simulink model "question5sigma"  (R2022b)
settings: Solver=ode4  StartTime=0.0  StopTime=10  FixedStep=0.0001  MaxStep=0.0001  RelTol=1e-3
values from neighbouring files (symbols this model uses):
  A = [a-b, 0.5-c; 0, 1]    [A2_1_2_graph.m]    (also in A2_1_2_val.m; A2_4_1.m = [a-bl, 0.5-c; 0, 1]; A2_4_3.m = [a-bl, 0.5-c; 0, 1]; A2_4_31.m = [a-bl, 0.5-c; 0, 1])
  B = [0; 1]    [A2_1_2_graph.m]    (also in A2_1_2_val.m; A2_4_1.m; A2_4_3.m; A2_4_31.m)
  C = eye(2)    [A2_5_1.m]
  D = zeros(2,1)    [A2_5_1.m]
settings Model: Creator=long  LastModifiedBy=munjunhwi
settings SolverCC: AlgebraicLoopSolver=TrustRegion
settings DebuggingCC: UnconnectedInputMsg=warning  UnconnectedOutputMsg=warning  UnconnectedLineMsg=warning  SFMachineParentedDataDiag=warning
settings ModelReferenceCC: EnableRefExpFcnMdlSchedulingChecks=on
settings RTWCC: DLArmComputeVersion=19.05

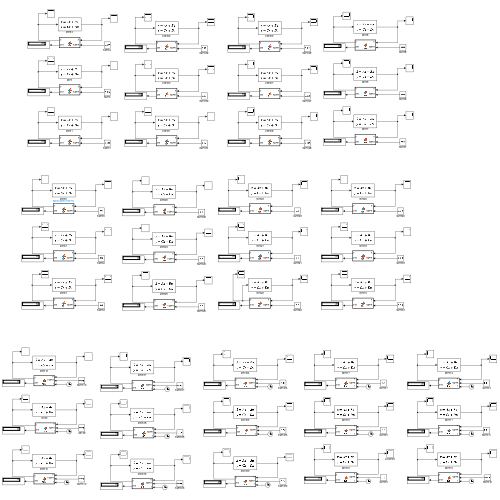
[thumbnail: Simulink's stored preview of the top-level diagram]
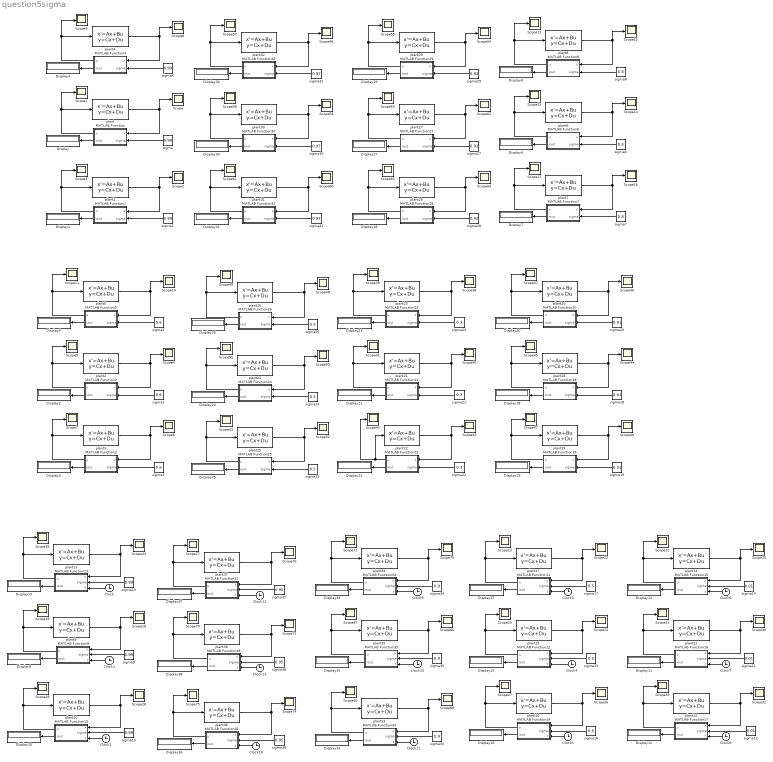
== system question5sigma ==
  Clock{,1..14} (15 alike) : Clock
  Display{,1..38} (39 alike) : Display
  MATLAB Function : MATLAB Function  TreatAsAtomicUnit=on
  MATLAB Function1 : MATLAB Function  TreatAsAtomicUnit=on
  MATLAB Function10 : MATLAB Function  TreatAsAtomicUnit=on
  MATLAB Function11 : MATLAB Function  TreatAsAtomicUnit=on
  MATLAB Function12 : MATLAB Function  TreatAsAtomicUnit=on
  MATLAB Function13 : MATLAB Function  TreatAsAtomicUnit=on
  MATLAB Function14 : MATLAB Function  TreatAsAtomicUnit=on
  MATLAB Function15 : MATLAB Function  TreatAsAtomicUnit=on
  MATLAB Function16 : MATLAB Function  TreatAsAtomicUnit=on
  MATLAB Function17 : MATLAB Function  TreatAsAtomicUnit=on
  MATLAB Function18 : MATLAB Function  TreatAsAtomicUnit=on
  MATLAB Function19 : MATLAB Function  TreatAsAtomicUnit=on
  MATLAB Function2 : MATLAB Function  TreatAsAtomicUnit=on
  MATLAB Function20 : MATLAB Function  TreatAsAtomicUnit=on
  MATLAB Function21 : MATLAB Function  TreatAsAtomicUnit=on
  MATLAB Function22 : MATLAB Function  TreatAsAtomicUnit=on
  MATLAB Function23 : MATLAB Function  TreatAsAtomicUnit=on
  MATLAB Function24 : MATLAB Function  TreatAsAtomicUnit=on
  MATLAB Function25 : MATLAB Function  TreatAsAtomicUnit=on
  MATLAB Function26 : MATLAB Function  TreatAsAtomicUnit=on
  MATLAB Function27 : MATLAB Function  TreatAsAtomicUnit=on
  MATLAB Function28 : MATLAB Function  TreatAsAtomicUnit=on
  MATLAB Function29 : MATLAB Function  TreatAsAtomicUnit=on
  MATLAB Function3 : MATLAB Function  TreatAsAtomicUnit=on
  MATLAB Function30 : MATLAB Function  TreatAsAtomicUnit=on
  MATLAB Function31 : MATLAB Function  TreatAsAtomicUnit=on
  MATLAB Function32 : MATLAB Function  TreatAsAtomicUnit=on
  MATLAB Function33 : MATLAB Function  TreatAsAtomicUnit=on
  MATLAB Function34 : MATLAB Function  TreatAsAtomicUnit=on
  MATLAB Function35 : MATLAB Function  TreatAsAtomicUnit=on
  MATLAB Function36 : MATLAB Function  TreatAsAtomicUnit=on
  MATLAB Function37 : MATLAB Function  TreatAsAtomicUnit=on
  MATLAB Function38 : MATLAB Function  TreatAsAtomicUnit=on
  MATLAB Function4 : MATLAB Function  TreatAsAtomicUnit=on
  MATLAB Function5 : MATLAB Function  TreatAsAtomicUnit=on
  MATLAB Function6 : MATLAB Function  TreatAsAtomicUnit=on
  MATLAB Function7 : MATLAB Function  TreatAsAtomicUnit=on
  MATLAB Function8 : MATLAB Function  TreatAsAtomicUnit=on
  MATLAB Function9 : MATLAB Function  TreatAsAtomicUnit=on
  Scope{,1..77} (78 alike) : Scope
  plant{,2,6,9,11,15,18,21,24,27,30,35,38} (13 alike) : StateSpace  A=A  B=B  C=C  D=D  InitialCondition=[10;10]
  plant{1,3,7,10,12,16,19,22,25,28,31,33,36} (13 alike) : StateSpace  A=A  B=B  C=C  D=D  InitialCondition=[1;0]
  plant{4..5,8,13..14,17,20,23,26,29,32,34,37} (13 alike) : StateSpace  A=A  B=B  C=C  D=D  InitialCondition=[100;150]
  sigma{,1,4,9..10,13} (6 alike) : Constant  Value=0.99
  sigma{11..12,14,18..20} (6 alike) : Constant  Value=0.01
  sigma{15..17,24..26} (6 alike) : Constant  Value=0.5
  sigma2 : Constant  Value=0.6
  sigma21 : Constant  Value=0.3
  sigma22 : Constant  Value=0.3
  sigma23 : Constant  Value=0.3
  sigma27 : Constant  Value=0.92
  sigma28 : Constant  Value=0.92
  sigma29 : Constant  Value=0.92
  sigma3 : Constant  Value=0.6
  sigma30 : Constant  Value=0.97
  sigma31 : Constant  Value=0.97
  sigma32 : Constant  Value=0.97
  sigma33 : Constant  Value=0.9
  sigma34 : Constant  Value=0.9
  sigma35 : Constant  Value=0.9
  sigma36 : Constant  Value=0.95
  sigma37 : Constant  Value=0.95
  sigma38 : Constant  Value=0.95
  sigma5 : Constant  Value=0.6
  sigma6 : Constant  Value=0.8
  sigma7 : Constant  Value=0.8
  sigma8 : Constant  Value=0.8
  wires:
  sigma/1 -> MATLAB Function/2(sigma)
  plant/1 -> MATLAB Function/1(x), Scope/1
  MATLAB Function/1(u) -> Scope1/1, plant/1
  MATLAB Function/2(iout) -> Display/1
  MATLAB Function1/2(iout) -> Display1/1
  MATLAB Function1/1(u) -> Scope3/1, plant1/1
  sigma1/1 -> MATLAB Function1/2(sigma)
  plant1/1 -> MATLAB Function1/1(x), Scope2/1
  MATLAB Function2/2(iout) -> Display2/1
  MATLAB Function2/1(u) -> Scope5/1, plant2/1
  sigma2/1 -> MATLAB Function2/2(sigma)
  plant2/1 -> MATLAB Function2/1(x), Scope4/1
  MATLAB Function3/2(iout) -> Display3/1
  MATLAB Function3/1(u) -> Scope7/1, plant3/1
  sigma3/1 -> MATLAB Function3/2(sigma)
  plant3/1 -> MATLAB Function3/1(x), Scope6/1
  sigma5/1 -> MATLAB Function5/2(sigma)
  MATLAB Function5/1(u) -> Scope11/1, plant5/1
  MATLAB Function4/2(iout) -> Display4/1
  MATLAB Function4/1(u) -> Scope9/1, plant4/1
  sigma4/1 -> MATLAB Function4/2(sigma)
  plant5/1 -> MATLAB Function5/1(x), Scope10/1
  MATLAB Function5/2(iout) -> Display5/1
  plant4/1 -> MATLAB Function4/1(x), Scope8/1
  sigma6/1 -> MATLAB Function6/2(sigma)
  MATLAB Function6/1(u) -> Scope15/1, plant6/1
  plant6/1 -> MATLAB Function6/1(x), Scope14/1
  MATLAB Function8/1(u) -> Scope13/1, plant8/1
  MATLAB Function8/2(iout) -> Display8/1
  plant8/1 -> MATLAB Function8/1(x), Scope12/1
  MATLAB Function6/2(iout) -> Display6/1
  sigma8/1 -> MATLAB Function8/2(sigma)
  sigma7/1 -> MATLAB Function7/2(sigma)
  MATLAB Function7/1(u) -> Scope17/1, plant7/1
  plant7/1 -> MATLAB Function7/1(x), Scope16/1
  MATLAB Function7/2(iout) -> Display7/1
  sigma11/1 -> MATLAB Function16/2(sigma)
  MATLAB Function16/1(u) -> Scope31/1, plant11/1
  plant11/1 -> MATLAB Function16/1(x), Scope30/1
  MATLAB Function10/2(iout) -> Display10/1
  sigma10/1 -> MATLAB Function10/2(sigma)
  plant10/1 -> MATLAB Function10/1(x), Scope28/1
  MATLAB Function15/1(u) -> Scope21/1, plant14/1
  MATLAB Function13/2(iout) -> Display13/1
  MATLAB Function13/1(u) -> Scope35/1, plant13/1
  plant14/1 -> MATLAB Function15/1(x), Scope20/1
  MATLAB Function16/2(iout) -> Display11/1
  MATLAB Function17/1(u) -> Scope33/1, plant12/1
  sigma12/1 -> MATLAB Function17/2(sigma)
  MATLAB Function17/2(iout) -> Display12/1
  plant12/1 -> MATLAB Function17/1(x), Scope32/1
  MATLAB Function14/2(iout) -> Display16/1
  plant16/1 -> MATLAB Function14/1(x), Scope26/1
  MATLAB Function12/2(iout) -> Display15/1
  sigma16/1 -> MATLAB Function14/2(sigma)
  plant17/1 -> MATLAB Function11/1(x), Scope22/1
  sigma14/1 -> MATLAB Function15/2(sigma)
  MATLAB Function14/1(u) -> Scope27/1, plant16/1
  MATLAB Function10/1(u) -> Scope29/1, plant10/1
  plant15/1 -> MATLAB Function12/1(x), Scope24/1
  MATLAB Function12/1(u) -> Scope25/1, plant15/1
  sigma13/1 -> MATLAB Function13/2(sigma)
  MATLAB Function11/2(iout) -> Display17/1
  MATLAB Function11/1(u) -> Scope23/1, plant17/1
  sigma17/1 -> MATLAB Function11/2(sigma)
  MATLAB Function9/1(u) -> Scope19/1, plant9/1
  MATLAB Function9/2(iout) -> Display9/1
  MATLAB Function15/2(iout) -> Display14/1
  sigma9/1 -> MATLAB Function9/2(sigma)
  plant9/1 -> MATLAB Function9/1(x), Scope18/1
  sigma15/1 -> MATLAB Function12/2(sigma)
  plant13/1 -> MATLAB Function13/1(x), Scope34/1
  Clock/1 -> MATLAB Function13/3(t)
  Clock1/1 -> MATLAB Function9/3(t)
  Clock2/1 -> MATLAB Function10/3(t)
  Clock3/1 -> MATLAB Function11/3(t)
  Clock4/1 -> MATLAB Function12/3(t)
  Clock5/1 -> MATLAB Function14/3(t)
  Clock6/1 -> MATLAB Function15/3(t)
  Clock7/1 -> MATLAB Function16/3(t)
  Clock8/1 -> MATLAB Function17/3(t)
  MATLAB Function18/2(iout) -> Display18/1
  MATLAB Function23/1(u) -> Scope39/1, plant23/1
  MATLAB Function22/2(iout) -> Display22/1
  MATLAB Function22/1(u) -> Scope43/1, plant22/1
  sigma22/1 -> MATLAB Function22/2(sigma)
  MATLAB Function23/2(iout) -> Display23/1
  sigma20/1 -> MATLAB Function20/2(sigma)
  plant23/1 -> MATLAB Function23/1(x), Scope38/1
  sigma23/1 -> MATLAB Function23/2(sigma)
  MATLAB Function19/2(iout) -> Display19/1
  MATLAB Function18/1(u) -> Scope45/1, plant18/1
  sigma18/1 -> MATLAB Function18/2(sigma)
  MATLAB Function20/1(u) -> Scope37/1, plant20/1
  plant18/1 -> MATLAB Function18/1(x), Scope44/1
  MATLAB Function20/2(iout) -> Display20/1
  plant20/1 -> MATLAB Function20/1(x), Scope36/1
  plant21/1 -> MATLAB Function21/1(x), Scope40/1
  MATLAB Function21/2(iout) -> Display21/1
  MATLAB Function21/1(u) -> Scope41/1, plant21/1
  plant19/1 -> MATLAB Function19/1(x), Scope46/1
  MATLAB Function19/1(u) -> Scope47/1, plant19/1
  plant22/1 -> MATLAB Function22/1(x), Scope42/1
  sigma19/1 -> MATLAB Function19/2(sigma)
  sigma21/1 -> MATLAB Function21/2(sigma)
  MATLAB Function26/1(u) -> Scope49/1, plant26/1
  MATLAB Function25/1(u) -> Scope53/1, plant25/1
  MATLAB Function24/2(iout) -> Display24/1
  sigma26/1 -> MATLAB Function26/2(sigma)
  sigma25/1 -> MATLAB Function25/2(sigma)
  plant26/1 -> MATLAB Function26/1(x), Scope48/1
  MATLAB Function26/2(iout) -> Display26/1
  MATLAB Function24/1(u) -> Scope51/1, plant24/1
  plant24/1 -> MATLAB Function24/1(x), Scope50/1
  MATLAB Function25/2(iout) -> Display25/1
  plant25/1 -> MATLAB Function25/1(x), Scope52/1
  sigma24/1 -> MATLAB Function24/2(sigma)
  MATLAB Function27/2(iout) -> Display27/1
  MATLAB Function32/1(u) -> Scope57/1, plant32/1
  MATLAB Function31/2(iout) -> Display31/1
  MATLAB Function31/1(u) -> Scope61/1, plant31/1
  sigma31/1 -> MATLAB Function31/2(sigma)
  MATLAB Function32/2(iout) -> Display32/1
  sigma29/1 -> MATLAB Function29/2(sigma)
  plant32/1 -> MATLAB Function32/1(x), Scope56/1
  sigma32/1 -> MATLAB Function32/2(sigma)
  MATLAB Function28/2(iout) -> Display28/1
  MATLAB Function27/1(u) -> Scope63/1, plant27/1
  sigma27/1 -> MATLAB Function27/2(sigma)
  MATLAB Function29/1(u) -> Scope55/1, plant29/1
  plant27/1 -> MATLAB Function27/1(x), Scope62/1
  MATLAB Function29/2(iout) -> Display29/1
  plant29/1 -> MATLAB Function29/1(x), Scope54/1
  plant30/1 -> MATLAB Function30/1(x), Scope58/1
  MATLAB Function30/2(iout) -> Display30/1
  MATLAB Function30/1(u) -> Scope59/1, plant30/1
  plant28/1 -> MATLAB Function28/1(x), Scope64/1
  MATLAB Function28/1(u) -> Scope65/1, plant28/1
  plant31/1 -> MATLAB Function31/1(x), Scope60/1
  sigma28/1 -> MATLAB Function28/2(sigma)
  sigma30/1 -> MATLAB Function30/2(sigma)
  MATLAB Function33/2(iout) -> Display33/1
  sigma33/1 -> MATLAB Function33/2(sigma)
  MATLAB Function35/2(iout) -> Display35/1
  MATLAB Function33/1(u) -> Scope69/1, plant33/1
  plant35/1 -> MATLAB Function35/1(x), Scope66/1
  MATLAB Function35/1(u) -> Scope67/1, plant35/1
  sigma34/1 -> MATLAB Function34/2(sigma)
  MATLAB Function34/2(iout) -> Display34/1
  sigma35/1 -> MATLAB Function35/2(sigma)
  MATLAB Function34/1(u) -> Scope71/1, plant34/1
  plant33/1 -> MATLAB Function33/1(x), Scope68/1
  plant34/1 -> MATLAB Function34/1(x), Scope70/1
  Clock9/1 -> MATLAB Function34/3(t)
  Clock10/1 -> MATLAB Function35/3(t)
  Clock11/1 -> MATLAB Function33/3(t)
  MATLAB Function36/2(iout) -> Display36/1
  sigma36/1 -> MATLAB Function36/2(sigma)
  MATLAB Function38/2(iout) -> Display38/1
  MATLAB Function36/1(u) -> Scope75/1, plant36/1
  plant38/1 -> MATLAB Function38/1(x), Scope72/1
  MATLAB Function38/1(u) -> Scope73/1, plant38/1
  sigma37/1 -> MATLAB Function37/2(sigma)
  MATLAB Function37/2(iout) -> Display37/1
  sigma38/1 -> MATLAB Function38/2(sigma)
  MATLAB Function37/1(u) -> Scope77/1, plant37/1
  plant36/1 -> MATLAB Function36/1(x), Scope74/1
  plant37/1 -> MATLAB Function37/1(x), Scope76/1
  Clock12/1 -> MATLAB Function37/3(t)
  Clock13/1 -> MATLAB Function38/3(t)
  Clock14/1 -> MATLAB Function36/3(t)

== matlab function question5sigma/MATLAB Function10 ==
  settings: updateMethod=DISCRETE
  data: x input; u output; sigma input; iout output; t input
function [u,iout]= fcn(x,sigma,t)
    persistent uk xk i;
    k1=zeros(1,2);
    A=zeros(2);
    B=zeros(2,1);
    P=zeros(2);
    Q=zeros(2);
    coder.extrinsic('evalin');
    A = evalin('base', 'A'); 
    B = evalin('base', 'B'); 
    P = evalin('base', 'P'); 
    Q = evalin('base', 'Q'); 
    k1 = evalin('base', 'k1'); 
    
    
    if isempty(uk)||isempty(xk)
        i=0;
        xk = x;
        uk=-k1*x;
    end

    
    if rem(t,0.2174)==0
        if [x' xk']*[A'*P+P*A+sigma*Q -P*B*k1;-(B*k1)'*P zeros(2)]*[x;xk]>=0
            i = i+1;
            uk = -k1*x;
            xk = x;
        end
    end

    u=uk;
    iout=i;
end

== matlab function question5sigma/MATLAB Function11 ==
  settings: updateMethod=DISCRETE
  data: x input; u output; sigma input; iout output; t input
function [u,iout]= fcn(x,sigma,t)
    persistent uk xk i;
    k1=zeros(1,2);
    A=zeros(2);
    B=zeros(2,1);
    P=zeros(2);
    Q=zeros(2);
    coder.extrinsic('evalin');
    A = evalin('base', 'A'); 
    B = evalin('base', 'B'); 
    P = evalin('base', 'P'); 
    Q = evalin('base', 'Q'); 
    k1 = evalin('base', 'k1'); 
    
    
    if isempty(uk)||isempty(xk)
        i=0;
        xk = x;
        uk=-k1*x;
    end

    
    if rem(t,0.2174)==0
        if [x' xk']*[A'*P+P*A+sigma*Q -P*B*k1;-(B*k1)'*P zeros(2)]*[x;xk]>=0
            i = i+1;
            uk = -k1*x;
            xk = x;
        end
    end

    u=uk;
    iout=i;
end

== matlab function question5sigma/MATLAB Function13 ==
  settings: updateMethod=DISCRETE
  data: x input; u output; sigma input; iout output; t input
function [u,iout]= fcn(x,sigma,t)
    persistent uk xk i;
    k1=zeros(1,2);
    A=zeros(2);
    B=zeros(2,1);
    P=zeros(2);
    Q=zeros(2);
    coder.extrinsic('evalin');
    A = evalin('base', 'A'); 
    B = evalin('base', 'B'); 
    P = evalin('base', 'P'); 
    Q = evalin('base', 'Q'); 
    k1 = evalin('base', 'k1'); 
    
    
    if isempty(uk)||isempty(xk)
        i=0;
        xk = x;
        uk=-k1*x;
    end

    
    if rem(t,0.2174)==0 %sampling time 0.0035
        if [x' xk']*[A'*P+P*A+sigma*Q -P*B*k1;-(B*k1)'*P zeros(2)]*[x;xk]>=0
            i = i+1;
            uk = -k1*x;
            xk = x;
        end
    end

    u=uk;
    iout=i;
end

== matlab function question5sigma/MATLAB Function12 ==
  settings: updateMethod=DISCRETE
  data: x input; u output; sigma input; iout output; t input
function [u,iout]= fcn(x,sigma,t)
    persistent uk xk i;
    k1=zeros(1,2);
    A=zeros(2);
    B=zeros(2,1);
    P=zeros(2);
    Q=zeros(2);
    coder.extrinsic('evalin');
    A = evalin('base', 'A'); 
    B = evalin('base', 'B'); 
    P = evalin('base', 'P'); 
    Q = evalin('base', 'Q'); 
    k1 = evalin('base', 'k1'); 
    
    
    if isempty(uk)||isempty(xk)
        i=0;
        xk = x;
        uk=-k1*x;
    end

    
    if rem(t,0.2174)==0
        if [x' xk']*[A'*P+P*A+sigma*Q -P*B*k1;-(B*k1)'*P zeros(2)]*[x;xk]>=0
            i = i+1;
            uk = -k1*x;
            xk = x;
        end
    end

    u=uk;
    iout=i;
end

== matlab function question5sigma/MATLAB Function14 ==
  settings: updateMethod=DISCRETE
  data: x input; u output; sigma input; iout output; t input
function [u,iout]= fcn(x,sigma,t)
    persistent uk xk i;
    k1=zeros(1,2);
    A=zeros(2);
    B=zeros(2,1);
    P=zeros(2);
    Q=zeros(2);
    coder.extrinsic('evalin');
    A = evalin('base', 'A'); 
    B = evalin('base', 'B'); 
    P = evalin('base', 'P'); 
    Q = evalin('base', 'Q'); 
    k1 = evalin('base', 'k1'); 
    
    
    if isempty(uk)||isempty(xk)
        i=0;
        xk = x;
        uk=-k1*x;
    end

    
    if rem(t,0.2174)==0
        if [x' xk']*[A'*P+P*A+sigma*Q -P*B*k1;-(B*k1)'*P zeros(2)]*[x;xk]>=0
            i = i+1;
            uk = -k1*x;
            xk = x;
        end
    end

    u=uk;
    iout=i;
end

== matlab function question5sigma/MATLAB Function15 ==
  settings: updateMethod=DISCRETE
  data: x input; u output; sigma input; iout output; t input
function [u,iout]= fcn(x,sigma,t)
    persistent uk xk i;
    k1=zeros(1,2);
    A=zeros(2);
    B=zeros(2,1);
    P=zeros(2);
    Q=zeros(2);
    coder.extrinsic('evalin');
    A = evalin('base', 'A'); 
    B = evalin('base', 'B'); 
    P = evalin('base', 'P'); 
    Q = evalin('base', 'Q'); 
    k1 = evalin('base', 'k1'); 
    
    
    if isempty(uk)||isempty(xk)
        i=0;
        xk = x;
        uk=-k1*x;
    end

    
    if rem(t,0.2174)==0
        if [x' xk']*[A'*P+P*A+sigma*Q -P*B*k1;-(B*k1)'*P zeros(2)]*[x;xk]>=0
            i = i+1;
            uk = -k1*x;
            xk = x;
        end
    end

    u=uk;
    iout=i;
end

== matlab function question5sigma/MATLAB Function1 ==
  settings: updateMethod=DISCRETE
  data: x input; u output; sigma input; iout output
function [u,iout]= fcn(x,sigma)
    persistent uk xk i;
    k1=zeros(1,2);
    A=zeros(2);
    B=zeros(2,1);
    P=zeros(2);
    Q=zeros(2);
    coder.extrinsic('evalin');
    A = evalin('base', 'A'); 
    B = evalin('base', 'B'); 
    P = evalin('base', 'P'); 
    Q = evalin('base', 'Q'); 
    k1 = evalin('base', 'k1'); 
    
    
    if isempty(uk)||isempty(xk)
        i=0;
        xk = x;
        uk=-k1*x;
    end

    if [x' xk']*[A'*P+P*A+sigma*Q -P*B*k1;-(B*k1)'*P zeros(2)]*[x;xk]>=0
        i = i+1;
        uk = -k1*x;
        xk = x;
    end

    u=uk;
    iout=i;
end

== matlab function question5sigma/MATLAB Function16 ==
  settings: updateMethod=DISCRETE
  data: x input; u output; sigma input; iout output; t input
function [u,iout]= fcn(x,sigma,t)
    persistent uk xk i;
    k1=zeros(1,2);
    A=zeros(2);
    B=zeros(2,1);
    P=zeros(2);
    Q=zeros(2);
    coder.extrinsic('evalin');
    A = evalin('base', 'A'); 
    B = evalin('base', 'B'); 
    P = evalin('base', 'P'); 
    Q = evalin('base', 'Q'); 
    k1 = evalin('base', 'k1'); 
    
    
    if isempty(uk)||isempty(xk)
        i=0;
        xk = x;
        uk=-k1*x;
    end

    
    if rem(t,0.2174)==0
        if [x' xk']*[A'*P+P*A+sigma*Q -P*B*k1;-(B*k1)'*P zeros(2)]*[x;xk]>=0
            i = i+1;
            uk = -k1*x;
            xk = x;
        end
    end

    u=uk;
    iout=i;
end

== matlab function question5sigma/MATLAB Function17 ==
  settings: updateMethod=DISCRETE
  data: x input; u output; sigma input; iout output; t input
function [u,iout]= fcn(x,sigma,t)
    persistent uk xk i;
    k1=zeros(1,2);
    A=zeros(2);
    B=zeros(2,1);
    P=zeros(2);
    Q=zeros(2);
    coder.extrinsic('evalin');
    A = evalin('base', 'A'); 
    B = evalin('base', 'B'); 
    P = evalin('base', 'P'); 
    Q = evalin('base', 'Q'); 
    k1 = evalin('base', 'k1'); 
    
    
    if isempty(uk)||isempty(xk)
        i=0;
        xk = x;
        uk=-k1*x;
    end

    
    if rem(t,0.2174)==0
        if [x' xk']*[A'*P+P*A+sigma*Q -P*B*k1;-(B*k1)'*P zeros(2)]*[x;xk]>=0
            i = i+1;
            uk = -k1*x;
            xk = x;
        end
    end

    u=uk;
    iout=i;
end

== matlab function question5sigma/MATLAB Function18 ==
  settings: updateMethod=DISCRETE
  data: x input; u output; sigma input; iout output
function [u,iout]= fcn(x,sigma)
    persistent uk xk i;
    k1=zeros(1,2);
    A=zeros(2);
    B=zeros(2,1);
    P=zeros(2);
    Q=zeros(2);
    coder.extrinsic('evalin');
    A = evalin('base', 'A'); 
    B = evalin('base', 'B'); 
    P = evalin('base', 'P'); 
    Q = evalin('base', 'Q'); 
    k1 = evalin('base', 'k1'); 
    
    
    if isempty(uk)||isempty(xk)
        i=0;
        xk = x;
        uk=-k1*x;
    end

    if [x' xk']*[A'*P+P*A+sigma*Q -P*B*k1;-(B*k1)'*P zeros(2)]*[x;xk]>=0
        i = i+1;
        uk = -k1*x;
        xk = x;
    end

    u=uk;
    iout=i;
end

== matlab function question5sigma/MATLAB Function19 ==
  settings: updateMethod=DISCRETE
  data: x input; u output; sigma input; iout output
function [u,iout]= fcn(x,sigma)
    persistent uk xk i;
    k1=zeros(1,2);
    A=zeros(2);
    B=zeros(2,1);
    P=zeros(2);
    Q=zeros(2);
    coder.extrinsic('evalin');
    A = evalin('base', 'A'); 
    B = evalin('base', 'B'); 
    P = evalin('base', 'P'); 
    Q = evalin('base', 'Q'); 
    k1 = evalin('base', 'k1'); 
    
    
    if isempty(uk)||isempty(xk)
        i=0;
        xk = x;
        uk=-k1*x;
    end

    if [x' xk']*[A'*P+P*A+sigma*Q -P*B*k1;-(B*k1)'*P zeros(2)]*[x;xk]>=0
        i = i+1;
        uk = -k1*x;
        xk = x;
    end

    u=uk;
    iout=i;
end

== matlab function question5sigma/MATLAB Function20 ==
  settings: updateMethod=DISCRETE
  data: x input; u output; sigma input; iout output
function [u,iout]= fcn(x,sigma)
    persistent uk xk i;
    k1=zeros(1,2);
    A=zeros(2);
    B=zeros(2,1);
    P=zeros(2);
    Q=zeros(2);
    coder.extrinsic('evalin');
    A = evalin('base', 'A'); 
    B = evalin('base', 'B'); 
    P = evalin('base', 'P'); 
    Q = evalin('base', 'Q'); 
    k1 = evalin('base', 'k1'); 
    
    
    if isempty(uk)||isempty(xk)
        i=0;
        xk = x;
        uk=-k1*x;
    end

    if [x' xk']*[A'*P+P*A+sigma*Q -P*B*k1;-(B*k1)'*P zeros(2)]*[x;xk]>=0
        i = i+1;
        uk = -k1*x;
        xk = x;
    end

    u=uk;
    iout=i;
end

== matlab function question5sigma/MATLAB Function21 ==
  settings: updateMethod=DISCRETE
  data: x input; u output; sigma input; iout output
function [u,iout]= fcn(x,sigma)
    persistent uk xk i;
    k1=zeros(1,2);
    A=zeros(2);
    B=zeros(2,1);
    P=zeros(2);
    Q=zeros(2);
    coder.extrinsic('evalin');
    A = evalin('base', 'A'); 
    B = evalin('base', 'B'); 
    P = evalin('base', 'P'); 
    Q = evalin('base', 'Q'); 
    k1 = evalin('base', 'k1'); 
    
    
    if isempty(uk)||isempty(xk)
        i=0;
        xk = x;
        uk=-k1*x;
    end

    if [x' xk']*[A'*P+P*A+sigma*Q -P*B*k1;-(B*k1)'*P zeros(2)]*[x;xk]>=0
        i = i+1;
        uk = -k1*x;
        xk = x;
    end

    u=uk;
    iout=i;
end

== matlab function question5sigma/MATLAB Function22 ==
  settings: updateMethod=DISCRETE
  data: x input; u output; sigma input; iout output
function [u,iout]= fcn(x,sigma)
    persistent uk xk i;
    k1=zeros(1,2);
    A=zeros(2);
    B=zeros(2,1);
    P=zeros(2);
    Q=zeros(2);
    coder.extrinsic('evalin');
    A = evalin('base', 'A'); 
    B = evalin('base', 'B'); 
    P = evalin('base', 'P'); 
    Q = evalin('base', 'Q'); 
    k1 = evalin('base', 'k1'); 
    
    
    if isempty(uk)||isempty(xk)
        i=0;
        xk = x;
        uk=-k1*x;
    end

    if [x' xk']*[A'*P+P*A+sigma*Q -P*B*k1;-(B*k1)'*P zeros(2)]*[x;xk]>=0
        i = i+1;
        uk = -k1*x;
        xk = x;
    end

    u=uk;
    iout=i;
end

== matlab function question5sigma/MATLAB Function23 ==
  settings: updateMethod=DISCRETE
  data: x input; u output; sigma input; iout output
function [u,iout]= fcn(x,sigma)
    persistent uk xk i;
    k1=zeros(1,2);
    A=zeros(2);
    B=zeros(2,1);
    P=zeros(2);
    Q=zeros(2);
    coder.extrinsic('evalin');
    A = evalin('base', 'A'); 
    B = evalin('base', 'B'); 
    P = evalin('base', 'P'); 
    Q = evalin('base', 'Q'); 
    k1 = evalin('base', 'k1'); 
    
    
    if isempty(uk)||isempty(xk)
        i=0;
        xk = x;
        uk=-k1*x;
    end

    if [x' xk']*[A'*P+P*A+sigma*Q -P*B*k1;-(B*k1)'*P zeros(2)]*[x;xk]>=0
        i = i+1;
        uk = -k1*x;
        xk = x;
    end

    u=uk;
    iout=i;
end

== matlab function question5sigma/MATLAB Function24 ==
  settings: updateMethod=DISCRETE
  data: x input; u output; sigma input; iout output
function [u,iout]= fcn(x,sigma)
    persistent uk xk i;
    k1=zeros(1,2);
    A=zeros(2);
    B=zeros(2,1);
    P=zeros(2);
    Q=zeros(2);
    coder.extrinsic('evalin');
    A = evalin('base', 'A'); 
    B = evalin('base', 'B'); 
    P = evalin('base', 'P'); 
    Q = evalin('base', 'Q'); 
    k1 = evalin('base', 'k1'); 
    
    
    if isempty(uk)||isempty(xk)
        i=0;
        xk = x;
        uk=-k1*x;
    end

    if [x' xk']*[A'*P+P*A+sigma*Q -P*B*k1;-(B*k1)'*P zeros(2)]*[x;xk]>=0
        i = i+1;
        uk = -k1*x;
        xk = x;
    end

    u=uk;
    iout=i;
end

== matlab function question5sigma/MATLAB Function ==
  settings: updateMethod=DISCRETE
  data: x input; u output; sigma input; iout output
function [u,iout]= fcn(x,sigma)
    persistent uk xk i;
    k1=zeros(1,2);
    A=zeros(2);
    B=zeros(2,1);
    P=zeros(2);
    Q=zeros(2);
    coder.extrinsic('evalin');
    A = evalin('base', 'A'); 
    B = evalin('base', 'B'); 
    P = evalin('base', 'P'); 
    Q = evalin('base', 'Q'); 
    k1 = evalin('base', 'k1'); 
    
    
    if isempty(uk)||isempty(xk)
        i=0;
        xk = x;
        uk=-k1*x;
    end

    if [x' xk']*[A'*P+P*A+sigma*Q -P*B*k1;-(B*k1)'*P zeros(2)]*[x;xk]>=0
        i = i+1;
        uk = -k1*x;
        xk = x;
    end

    u=uk;
    iout=i;
end

== matlab function question5sigma/MATLAB Function25 ==
  settings: updateMethod=DISCRETE
  data: x input; u output; sigma input; iout output
function [u,iout]= fcn(x,sigma)
    persistent uk xk i;
    k1=zeros(1,2);
    A=zeros(2);
    B=zeros(2,1);
    P=zeros(2);
    Q=zeros(2);
    coder.extrinsic('evalin');
    A = evalin('base', 'A'); 
    B = evalin('base', 'B'); 
    P = evalin('base', 'P'); 
    Q = evalin('base', 'Q'); 
    k1 = evalin('base', 'k1'); 
    
    
    if isempty(uk)||isempty(xk)
        i=0;
        xk = x;
        uk=-k1*x;
    end

    if [x' xk']*[A'*P+P*A+sigma*Q -P*B*k1;-(B*k1)'*P zeros(2)]*[x;xk]>=0
        i = i+1;
        uk = -k1*x;
        xk = x;
    end

    u=uk;
    iout=i;
end

== matlab function question5sigma/MATLAB Function26 ==
  settings: updateMethod=DISCRETE
  data: x input; u output; sigma input; iout output
function [u,iout]= fcn(x,sigma)
    persistent uk xk i;
    k1=zeros(1,2);
    A=zeros(2);
    B=zeros(2,1);
    P=zeros(2);
    Q=zeros(2);
    coder.extrinsic('evalin');
    A = evalin('base', 'A'); 
    B = evalin('base', 'B'); 
    P = evalin('base', 'P'); 
    Q = evalin('base', 'Q'); 
    k1 = evalin('base', 'k1'); 
    
    
    if isempty(uk)||isempty(xk)
        i=0;
        xk = x;
        uk=-k1*x;
    end

    if [x' xk']*[A'*P+P*A+sigma*Q -P*B*k1;-(B*k1)'*P zeros(2)]*[x;xk]>=0
        i = i+1;
        uk = -k1*x;
        xk = x;
    end

    u=uk;
    iout=i;
end

== matlab function question5sigma/MATLAB Function27 ==
  settings: updateMethod=DISCRETE
  data: x input; u output; sigma input; iout output
function [u,iout]= fcn(x,sigma)
    persistent uk xk i;
    k1=zeros(1,2);
    A=zeros(2);
    B=zeros(2,1);
    P=zeros(2);
    Q=zeros(2);
    coder.extrinsic('evalin');
    A = evalin('base', 'A'); 
    B = evalin('base', 'B'); 
    P = evalin('base', 'P'); 
    Q = evalin('base', 'Q'); 
    k1 = evalin('base', 'k1'); 
    
    
    if isempty(uk)||isempty(xk)
        i=0;
        xk = x;
        uk=-k1*x;
    end

    if [x' xk']*[A'*P+P*A+sigma*Q -P*B*k1;-(B*k1)'*P zeros(2)]*[x;xk]>=0
        i = i+1;
        uk = -k1*x;
        xk = x;
    end

    u=uk;
    iout=i;
end

== matlab function question5sigma/MATLAB Function28 ==
  settings: updateMethod=DISCRETE
  data: x input; u output; sigma input; iout output
function [u,iout]= fcn(x,sigma)
    persistent uk xk i;
    k1=zeros(1,2);
    A=zeros(2);
    B=zeros(2,1);
    P=zeros(2);
    Q=zeros(2);
    coder.extrinsic('evalin');
    A = evalin('base', 'A'); 
    B = evalin('base', 'B'); 
    P = evalin('base', 'P'); 
    Q = evalin('base', 'Q'); 
    k1 = evalin('base', 'k1'); 
    
    
    if isempty(uk)||isempty(xk)
        i=0;
        xk = x;
        uk=-k1*x;
    end

    if [x' xk']*[A'*P+P*A+sigma*Q -P*B*k1;-(B*k1)'*P zeros(2)]*[x;xk]>=0
        i = i+1;
        uk = -k1*x;
        xk = x;
    end

    u=uk;
    iout=i;
end

== matlab function question5sigma/MATLAB Function29 ==
  settings: updateMethod=DISCRETE
  data: x input; u output; sigma input; iout output
function [u,iout]= fcn(x,sigma)
    persistent uk xk i;
    k1=zeros(1,2);
    A=zeros(2);
    B=zeros(2,1);
    P=zeros(2);
    Q=zeros(2);
    coder.extrinsic('evalin');
    A = evalin('base', 'A'); 
    B = evalin('base', 'B'); 
    P = evalin('base', 'P'); 
    Q = evalin('base', 'Q'); 
    k1 = evalin('base', 'k1'); 
    
    
    if isempty(uk)||isempty(xk)
        i=0;
        xk = x;
        uk=-k1*x;
    end

    if [x' xk']*[A'*P+P*A+sigma*Q -P*B*k1;-(B*k1)'*P zeros(2)]*[x;xk]>=0
        i = i+1;
        uk = -k1*x;
        xk = x;
    end

    u=uk;
    iout=i;
end

== matlab function question5sigma/MATLAB Function30 ==
  settings: updateMethod=DISCRETE
  data: x input; u output; sigma input; iout output
function [u,iout]= fcn(x,sigma)
    persistent uk xk i;
    k1=zeros(1,2);
    A=zeros(2);
    B=zeros(2,1);
    P=zeros(2);
    Q=zeros(2);
    coder.extrinsic('evalin');
    A = evalin('base', 'A'); 
    B = evalin('base', 'B'); 
    P = evalin('base', 'P'); 
    Q = evalin('base', 'Q'); 
    k1 = evalin('base', 'k1'); 
    
    
    if isempty(uk)||isempty(xk)
        i=0;
        xk = x;
        uk=-k1*x;
    end

    if [x' xk']*[A'*P+P*A+sigma*Q -P*B*k1;-(B*k1)'*P zeros(2)]*[x;xk]>=0
        i = i+1;
        uk = -k1*x;
        xk = x;
    end

    u=uk;
    iout=i;
end

== matlab function question5sigma/MATLAB Function31 ==
  settings: updateMethod=DISCRETE
  data: x input; u output; sigma input; iout output
function [u,iout]= fcn(x,sigma)
    persistent uk xk i;
    k1=zeros(1,2);
    A=zeros(2);
    B=zeros(2,1);
    P=zeros(2);
    Q=zeros(2);
    coder.extrinsic('evalin');
    A = evalin('base', 'A'); 
    B = evalin('base', 'B'); 
    P = evalin('base', 'P'); 
    Q = evalin('base', 'Q'); 
    k1 = evalin('base', 'k1'); 
    
    
    if isempty(uk)||isempty(xk)
        i=0;
        xk = x;
        uk=-k1*x;
    end

    if [x' xk']*[A'*P+P*A+sigma*Q -P*B*k1;-(B*k1)'*P zeros(2)]*[x;xk]>=0
        i = i+1;
        uk = -k1*x;
        xk = x;
    end

    u=uk;
    iout=i;
end

== matlab function question5sigma/MATLAB Function32 ==
  settings: updateMethod=DISCRETE
  data: x input; u output; sigma input; iout output
function [u,iout]= fcn(x,sigma)
    persistent uk xk i;
    k1=zeros(1,2);
    A=zeros(2);
    B=zeros(2,1);
    P=zeros(2);
    Q=zeros(2);
    coder.extrinsic('evalin');
    A = evalin('base', 'A'); 
    B = evalin('base', 'B'); 
    P = evalin('base', 'P'); 
    Q = evalin('base', 'Q'); 
    k1 = evalin('base', 'k1'); 
    
    
    if isempty(uk)||isempty(xk)
        i=0;
        xk = x;
        uk=-k1*x;
    end

    if [x' xk']*[A'*P+P*A+sigma*Q -P*B*k1;-(B*k1)'*P zeros(2)]*[x;xk]>=0
        i = i+1;
        uk = -k1*x;
        xk = x;
    end

    u=uk;
    iout=i;
end

== matlab function question5sigma/MATLAB Function33 ==
  settings: updateMethod=DISCRETE
  data: x input; u output; sigma input; iout output; t input
function [u,iout]= fcn(x,sigma,t)
    persistent uk xk i;
    k1=zeros(1,2);
    A=zeros(2);
    B=zeros(2,1);
    P=zeros(2);
    Q=zeros(2);
    coder.extrinsic('evalin');
    A = evalin('base', 'A'); 
    B = evalin('base', 'B'); 
    P = evalin('base', 'P'); 
    Q = evalin('base', 'Q'); 
    k1 = evalin('base', 'k1'); 
    
    
    if isempty(uk)||isempty(xk)
        i=0;
        xk = x;
        uk=-k1*x;
    end

    
    if rem(t,0.2174)==0
        if [x' xk']*[A'*P+P*A+sigma*Q -P*B*k1;-(B*k1)'*P zeros(2)]*[x;xk]>=0
            i = i+1;
            uk = -k1*x;
            xk = x;
        end
    end

    u=uk;
    iout=i;
end

== matlab function question5sigma/MATLAB Function34 ==
  settings: updateMethod=DISCRETE
  data: x input; u output; sigma input; iout output; t input
function [u,iout]= fcn(x,sigma,t)
    persistent uk xk i;
    k1=zeros(1,2);
    A=zeros(2);
    B=zeros(2,1);
    P=zeros(2);
    Q=zeros(2);
    coder.extrinsic('evalin');
    A = evalin('base', 'A'); 
    B = evalin('base', 'B'); 
    P = evalin('base', 'P'); 
    Q = evalin('base', 'Q'); 
    k1 = evalin('base', 'k1'); 
    
    
    if isempty(uk)||isempty(xk)
        i=0;
        xk = x;
        uk=-k1*x;
    end

    
    if rem(t,0.2174)==0 %sampling time 0.0035
        if [x' xk']*[A'*P+P*A+sigma*Q -P*B*k1;-(B*k1)'*P zeros(2)]*[x;xk]>=0
            i = i+1;
            uk = -k1*x;
            xk = x;
        end
    end

    u=uk;
    iout=i;
end

== matlab function question5sigma/MATLAB Function2 ==
  settings: updateMethod=DISCRETE
  data: x input; u output; sigma input; iout output
function [u,iout]= fcn(x,sigma)
    persistent uk xk i;
    k1=zeros(1,2);
    A=zeros(2);
    B=zeros(2,1);
    P=zeros(2);
    Q=zeros(2);
    coder.extrinsic('evalin');
    A = evalin('base', 'A'); 
    B = evalin('base', 'B'); 
    P = evalin('base', 'P'); 
    Q = evalin('base', 'Q'); 
    k1 = evalin('base', 'k1'); 
    
    
    if isempty(uk)||isempty(xk)
        i=0;
        xk = x;
        uk=-k1*x;
    end

    if [x' xk']*[A'*P+P*A+sigma*Q -P*B*k1;-(B*k1)'*P zeros(2)]*[x;xk]>=0
        i = i+1;
        uk = -k1*x;
        xk = x;
    end

    u=uk;
    iout=i;
end

== matlab function question5sigma/MATLAB Function35 ==
  settings: updateMethod=DISCRETE
  data: x input; u output; sigma input; iout output; t input
function [u,iout]= fcn(x,sigma,t)
    persistent uk xk i;
    k1=zeros(1,2);
    A=zeros(2);
    B=zeros(2,1);
    P=zeros(2);
    Q=zeros(2);
    coder.extrinsic('evalin');
    A = evalin('base', 'A'); 
    B = evalin('base', 'B'); 
    P = evalin('base', 'P'); 
    Q = evalin('base', 'Q'); 
    k1 = evalin('base', 'k1'); 
    
    
    if isempty(uk)||isempty(xk)
        i=0;
        xk = x;
        uk=-k1*x;
    end

    
    if rem(t,0.2174)==0
        if [x' xk']*[A'*P+P*A+sigma*Q -P*B*k1;-(B*k1)'*P zeros(2)]*[x;xk]>=0
            i = i+1;
            uk = -k1*x;
            xk = x;
        end
    end

    u=uk;
    iout=i;
end

== matlab function question5sigma/MATLAB Function36 ==
  settings: updateMethod=DISCRETE
  data: x input; u output; sigma input; iout output; t input
function [u,iout]= fcn(x,sigma,t)
    persistent uk xk i;
    k1=zeros(1,2);
    A=zeros(2);
    B=zeros(2,1);
    P=zeros(2);
    Q=zeros(2);
    coder.extrinsic('evalin');
    A = evalin('base', 'A'); 
    B = evalin('base', 'B'); 
    P = evalin('base', 'P'); 
    Q = evalin('base', 'Q'); 
    k1 = evalin('base', 'k1'); 
    
    
    if isempty(uk)||isempty(xk)
        i=0;
        xk = x;
        uk=-k1*x;
    end

    
    if rem(t,0.2174)==0
        if [x' xk']*[A'*P+P*A+sigma*Q -P*B*k1;-(B*k1)'*P zeros(2)]*[x;xk]>=0
            i = i+1;
            uk = -k1*x;
            xk = x;
        end
    end

    u=uk;
    iout=i;
end

== matlab function question5sigma/MATLAB Function37 ==
  settings: updateMethod=DISCRETE
  data: x input; u output; sigma input; iout output; t input
function [u,iout]= fcn(x,sigma,t)
    persistent uk xk i;
    k1=zeros(1,2);
    A=zeros(2);
    B=zeros(2,1);
    P=zeros(2);
    Q=zeros(2);
    coder.extrinsic('evalin');
    A = evalin('base', 'A'); 
    B = evalin('base', 'B'); 
    P = evalin('base', 'P'); 
    Q = evalin('base', 'Q'); 
    k1 = evalin('base', 'k1'); 
    
    
    if isempty(uk)||isempty(xk)
        i=0;
        xk = x;
        uk=-k1*x;
    end

    
    if rem(t,0.2174)==0 %sampling time 0.0035
        if [x' xk']*[A'*P+P*A+sigma*Q -P*B*k1;-(B*k1)'*P zeros(2)]*[x;xk]>=0
            i = i+1;
            uk = -k1*x;
            xk = x;
        end
    end

    u=uk;
    iout=i;
end

== matlab function question5sigma/MATLAB Function38 ==
  settings: updateMethod=DISCRETE
  data: x input; u output; sigma input; iout output; t input
function [u,iout]= fcn(x,sigma,t)
    persistent uk xk i;
    k1=zeros(1,2);
    A=zeros(2);
    B=zeros(2,1);
    P=zeros(2);
    Q=zeros(2);
    coder.extrinsic('evalin');
    A = evalin('base', 'A'); 
    B = evalin('base', 'B'); 
    P = evalin('base', 'P'); 
    Q = evalin('base', 'Q'); 
    k1 = evalin('base', 'k1'); 
    
    
    if isempty(uk)||isempty(xk)
        i=0;
        xk = x;
        uk=-k1*x;
    end

    
    if rem(t,0.2174)==0
        if [x' xk']*[A'*P+P*A+sigma*Q -P*B*k1;-(B*k1)'*P zeros(2)]*[x;xk]>=0
            i = i+1;
            uk = -k1*x;
            xk = x;
        end
    end

    u=uk;
    iout=i;
end

== matlab function question5sigma/MATLAB Function3 ==
  settings: updateMethod=DISCRETE
  data: x input; u output; sigma input; iout output
function [u,iout]= fcn(x,sigma)
    persistent uk xk i;
    k1=zeros(1,2);
    A=zeros(2);
    B=zeros(2,1);
    P=zeros(2);
    Q=zeros(2);
    coder.extrinsic('evalin');
    A = evalin('base', 'A'); 
    B = evalin('base', 'B'); 
    P = evalin('base', 'P'); 
    Q = evalin('base', 'Q'); 
    k1 = evalin('base', 'k1'); 
    
    
    if isempty(uk)||isempty(xk)
        i=0;
        xk = x;
        uk=-k1*x;
    end

    if [x' xk']*[A'*P+P*A+sigma*Q -P*B*k1;-(B*k1)'*P zeros(2)]*[x;xk]>=0
        i = i+1;
        uk = -k1*x;
        xk = x;
    end

    u=uk;
    iout=i;
end

== matlab function question5sigma/MATLAB Function4 ==
  settings: updateMethod=DISCRETE
  data: x input; u output; sigma input; iout output
function [u,iout]= fcn(x,sigma)
    persistent uk xk i;
    k1=zeros(1,2);
    A=zeros(2);
    B=zeros(2,1);
    P=zeros(2);
    Q=zeros(2);
    coder.extrinsic('evalin');
    A = evalin('base', 'A'); 
    B = evalin('base', 'B'); 
    P = evalin('base', 'P'); 
    Q = evalin('base', 'Q'); 
    k1 = evalin('base', 'k1'); 
    
    
    if isempty(uk)||isempty(xk)
        i=0;
        xk = x;
        uk=-k1*x;
    end

    if [x' xk']*[A'*P+P*A+sigma*Q -P*B*k1;-(B*k1)'*P zeros(2)]*[x;xk]>=0
        i = i+1;
        uk = -k1*x;
        xk = x;
    end

    u=uk;
    iout=i;
end

== matlab function question5sigma/MATLAB Function5 ==
  settings: updateMethod=DISCRETE
  data: x input; u output; sigma input; iout output
function [u,iout]= fcn(x,sigma)
    persistent uk xk i;
    k1=zeros(1,2);
    A=zeros(2);
    B=zeros(2,1);
    P=zeros(2);
    Q=zeros(2);
    coder.extrinsic('evalin');
    A = evalin('base', 'A'); 
    B = evalin('base', 'B'); 
    P = evalin('base', 'P'); 
    Q = evalin('base', 'Q'); 
    k1 = evalin('base', 'k1'); 
    
    
    if isempty(uk)||isempty(xk)
        i=0;
        xk = x;
        uk=-k1*x;
    end

    if [x' xk']*[A'*P+P*A+sigma*Q -P*B*k1;-(B*k1)'*P zeros(2)]*[x;xk]>=0
        i = i+1;
        uk = -k1*x;
        xk = x;
    end

    u=uk;
    iout=i;
end

== matlab function question5sigma/MATLAB Function6 ==
  settings: updateMethod=DISCRETE
  data: x input; u output; sigma input; iout output
function [u,iout]= fcn(x,sigma)
    persistent uk xk i;
    k1=zeros(1,2);
    A=zeros(2);
    B=zeros(2,1);
    P=zeros(2);
    Q=zeros(2);
    coder.extrinsic('evalin');
    A = evalin('base', 'A'); 
    B = evalin('base', 'B'); 
    P = evalin('base', 'P'); 
    Q = evalin('base', 'Q'); 
    k1 = evalin('base', 'k1'); 
    
    
    if isempty(uk)||isempty(xk)
        i=0;
        xk = x;
        uk=-k1*x;
    end

    if [x' xk']*[A'*P+P*A+sigma*Q -P*B*k1;-(B*k1)'*P zeros(2)]*[x;xk]>=0
        i = i+1;
        uk = -k1*x;
        xk = x;
    end

    u=uk;
    iout=i;
end

== matlab function question5sigma/MATLAB Function7 ==
  settings: updateMethod=DISCRETE
  data: x input; u output; sigma input; iout output
function [u,iout]= fcn(x,sigma)
    persistent uk xk i;
    k1=zeros(1,2);
    A=zeros(2);
    B=zeros(2,1);
    P=zeros(2);
    Q=zeros(2);
    coder.extrinsic('evalin');
    A = evalin('base', 'A'); 
    B = evalin('base', 'B'); 
    P = evalin('base', 'P'); 
    Q = evalin('base', 'Q'); 
    k1 = evalin('base', 'k1'); 
    
    
    if isempty(uk)||isempty(xk)
        i=0;
        xk = x;
        uk=-k1*x;
    end

    if [x' xk']*[A'*P+P*A+sigma*Q -P*B*k1;-(B*k1)'*P zeros(2)]*[x;xk]>=0
        i = i+1;
        uk = -k1*x;
        xk = x;
    end

    u=uk;
    iout=i;
end

== matlab function question5sigma/MATLAB Function8 ==
  settings: updateMethod=DISCRETE
  data: x input; u output; sigma input; iout output
function [u,iout]= fcn(x,sigma)
    persistent uk xk i;
    k1=zeros(1,2);
    A=zeros(2);
    B=zeros(2,1);
    P=zeros(2);
    Q=zeros(2);
    coder.extrinsic('evalin');
    A = evalin('base', 'A'); 
    B = evalin('base', 'B'); 
    P = evalin('base', 'P'); 
    Q = evalin('base', 'Q'); 
    k1 = evalin('base', 'k1'); 
    
    
    if isempty(uk)||isempty(xk)
        i=0;
        xk = x;
        uk=-k1*x;
    end

    if [x' xk']*[A'*P+P*A+sigma*Q -P*B*k1;-(B*k1)'*P zeros(2)]*[x;xk]>=0
        i = i+1;
        uk = -k1*x;
        xk = x;
    end

    u=uk;
    iout=i;
end

== matlab function question5sigma/MATLAB Function9 ==
  settings: updateMethod=DISCRETE
  data: x input; u output; sigma input; iout output; t input
function [u,iout]= fcn(x,sigma,t)
    persistent uk xk i;
    k1=zeros(1,2);
    A=zeros(2);
    B=zeros(2,1);
    P=zeros(2);
    Q=zeros(2);
    coder.extrinsic('evalin');
    A = evalin('base', 'A'); 
    B = evalin('base', 'B'); 
    P = evalin('base', 'P'); 
    Q = evalin('base', 'Q'); 
    k1 = evalin('base', 'k1'); 
    
    
    if isempty(uk)||isempty(xk)
        i=0;
        xk = x;
        uk=-k1*x;
    end

    
    if rem(t,0.2174)==0
        if [x' xk']*[A'*P+P*A+sigma*Q -P*B*k1;-(B*k1)'*P zeros(2)]*[x;xk]>=0
            i = i+1;
            uk = -k1*x;
            xk = x;
        end
    end

    u=uk;
    iout=i;
end
